simulink model "LimitChecking_RunningMean"  (R2014a)
settings: Solver=FixedStepDiscrete  StartTime=0.0  StopTime=inf  FixedStep=SampleTime  RelTol=1e-3
InitFcn:
  | limit_runningmean = 0.125;
libraries: simulink x1, dspbuff3 x1, dspstat3 x1
settings Model: Creator=georg  LastModifiedBy=georg

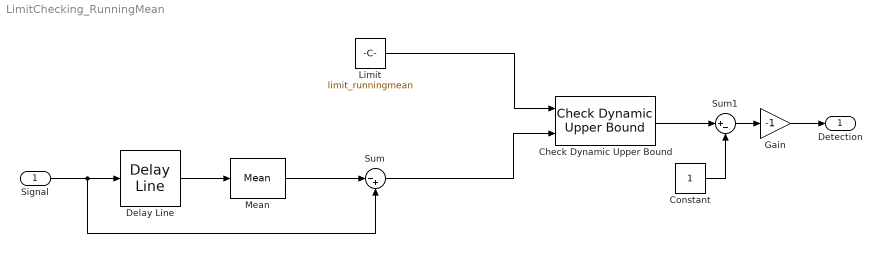
== system LimitChecking_RunningMean ==
  Signal : Inport
  Check Dynamic Upper Bound : simulink/Model Verification/Check Dynamic  Upper Bound  Description=sig < max  enabled=on  stopWhenAssertionFail=off  export=on  icon=graphic
  Constant : Constant
  Delay Line : dspbuff3/Delay Line  siz=3  ic=0  directfeed=off  enable_output=off  hold_output=off  TreatMby1Signals=One channel
  Gain : Gain  Gain=-1
  Limit : Constant  Value=limit_runningmean
  Mean : dspstat3/Mean  run=off  reset_popup=None  InputProcessing=Columns as channels (frame based)  directionMode=Entire input  dimension=1  treatSBRowAsCol=on  roiEnable=off  roiType=Rectangles  roiPortion=Entire ROI  roiOutput=Individual statistics for each ROI  roiFlag=off  outputDataTypeStr=Inherit: Same as accumulator  outputLastDataTypeStr=Inherit: Same as accumulator  outputMin=[]  outputMax=[]  roundingMode=Floor  overflowMode=off
  Sum : Sum  Inputs=|-+
  Sum1 : Sum  Inputs=|+-
  Detection : Outport  PortDimensions=1
  wires:
  Mean/1 -> Sum/1
  Check Dynamic Upper Bound/1 -> Sum1/1
  Sum/1 -> Check Dynamic Upper Bound/2
  Limit/1 -> Check Dynamic Upper Bound/1
  Constant/1 -> Sum1/2
  Sum1/1 -> Gain/1
  Gain/1 -> Detection/1
  Signal/1 -> Sum/2, Delay Line/1
  Delay Line/1 -> Mean/1
